simulink library "GenLib"  (R2019b)
settings: Solver=VariableStepAuto  StartTime=0.0  StopTime=10.0  RelTol=1e-3
undefined symbols (not defined in the file or in its folder): A, Ac, B, Bc, C, Cc, Dc, Dd, g, gcbh, I1_init, j, Mag_V0, np, nq, p, P0, PQext, Q0, sps_rtmsupport, Tp1, Tp2, Tq1, Tq2, Vbase, Vmin, Vnom
settings Model: Creator=haochen  LastModifiedBy=gdudgeon
settings DataIOCC: ReturnWorkspaceOutputs=off
settings OptimizationCC: LifeSpan=inf
settings DebuggingCC: SFExecutionAtInitializationDiag=none  ArithmeticOperatorsInVariantConditions=warning
settings SFSimCC: SimUseLocalCustomCode=off  CustomCodeUndefinedFunction=UseInterfaceOnly
settings RTWCC: RTWUseLocalCustomCode=off
settings CodeAppCC: StateflowObjectComments=on
settings ConfigComp: CovMetricSettings=dswe

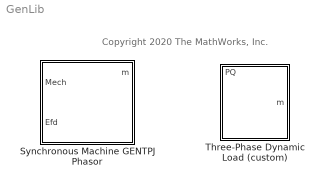
== system GenLib ==
  note: Copyright 2020 The MathWorks, Inc.
  Synchronous Machine GENTPJ Phasor : Subsystem  DialogController=POWERSYS.PowerSysDialog  LoadFcn=sps_rtmsupport('LoadFcn',gcbh);  StartFcn=sps_rtmsupport('StartFcn',gcbh);  StopFcn=sps_rtmsupport('StopFcn',gcbh);  mask(Synchronous Machine){PresetModel=No, MechanicalLoad=Mechanical power Pm, ShowDetailedParameters=on, RotorType=Salient-pole, Units=per unit fundamental parameters, MeasurementBus=off, NominalParameters=[ 187E6  13800   60], Stator=[ 2.85E-03  0.114  1.19  0.36 ], Field=[ 5.79E-04  0.114], Dampers2=[0.0652, 0.5134, 0.0287, 0.2553, 7.765e-3, 0.9167 ], Dampers1=[ 1.17E-02  0.182  1.97E-02  0.384 ], Mechanical=[ 3.7 0 20], PolePairs=20, InitialConditions=[ 0  0  0  0  0  0  0  0  1 ], SetSaturation=off, Saturation=[0.6404,0.7127,0.8441,0.9214,0.9956,1.082,1.19,1.316,1.457;0.7,0.7698,0.8872,0.9466,0.9969,1.046,1.1,1.151,1.201], LoadFlowParameters=[1,0,0,0,0], TsPowergui=0, TsBlock=-1, IterativeModel=Trapezoidal non iterative, IterativeDiscreteModel=Trapezoidal non iterative, BusType=PV, Pref=0, Qref=0, Qmin=-inf, Qmax=inf, PLF=0, QLF=0, Pnom=g.MBASE*1e6, Vnom=g.BUSV*1e3, fnom=60, Ra=p.ra, Xl=p.ll, Xd=p.ld, Xq=p.lq, Xdp=p.lpd, Xqp=p.lpq, Xdpp=p.lppd, Xqpp=p.lppq, Tdop=p.tpdo, Tqop=p.tpqo, Tdopp=p.tppdo, Tqopp=p.tppqo, SatOption=Quadratic, Ifd=[0 0.5 0.6 0.7 0.8 0.9 1 1.0562 1.1184 1.1985 1.2994 1.4576 1.6524 2.2234], Vag=[0 0.5 0.6 0.7 0.8 0.9 0.995 1.05 1.1 1.15 1.2 1.25 1.3 1.4], S10S12=[p.s1 p.s12], Kis=p.kis, SatOn=on, InputType=Mechanical power Pm, H=p.h, D=p.d}
      mask prompts: PresetModel "Preset  model:"; MechanicalLoad "Mechanical input:"; ShowDetailedParameters "Show detailed parameters"; RotorType "Rotor type:"; Units "Mask units:"; MeasurementBus "Use signal names to identify bus labels"; NominalParameters "Nominal power, line-to-line voltage and frequency [ Pn(VA)  Vn(Vrms)  fn(Hz) ]:"; Stator "Stator  [ Rs  Ll  Lmd  Lmq ] (pu):"; Field "Field  [ Rf  Llfd ] (pu):"; Dampers2 "Dampers  [ Rkd  Llkd  Rkq1  Llkq1  Rkq2  Llkq2 ] (pu):"; Dampers1 "Dampers  [ Rkd  Llkd  Rkq1  Llkq1 ] (pu):"; Mechanical "Inertia coeficient, friction factor, pole pairs [ H(s)  F(pu)  p() ]:"; PolePairs "Pole pairs p ():"; InitialConditions "Initial conditions [ dw(%)  th(deg)  ia,ib,ic(pu)  pha,phb,phc(deg)  Vf(pu) ]:"; SetSaturation "Simulate saturation"; Saturation "[ ifd; vt] (pu):"; LoadFlowParameters "Load Flow:   [Bus Type, Active Power,  UAB, phase of UAN ]"; TsPowergui "Sample time of powergui block:"; TsBlock "Sample time (-1 for inherited):"; IterativeDiscreteModel "Discrete solver model"; BusType "Generator type:"; Pref "Active power generation P (W):"; Qref "Reactive power generation Q (var):"; Qmin "Minimum reactive power Qmin (var):"; Qmax "Maximum reactive power Qmax (var):"; PLF "Load flow solution:  P_LF (W):"; QLF "Load flow solution:  Q_LF (var):"; Pnom "Nominal power (VA):"; Vnom "Nominal line-to-line voltage (Vrms):"; fnom "Nominal frequency (Hz):"; Ra "Stator resistance Ra:"; Xl "Stator leakage reactance Xl:"; Xd "d-axis reactance Xd:"; Xq "q-axis reactance Xq:"; Xdp "d-axis transient reactance Xd':"; Xqp "q-axis transient reactance Xq':"; Xdpp "d-axis subtransient reactance Xd'':"; Xqpp "q-axis subtransient reactance Xq'':"; Tdop "d-axis transient open-circuit time constant Tdo' (s):"; Tqop "q-axis transient open-circuit time constant Tqo' (s):"; Tdopp "d-axis subtransient open-circuit time constant Tdo''(s):"; Tqopp "q-axis subtransient open-circuit time constant Tqo''(s):"; SatOption "Option:"; Ifd "Field current saturation data (non-reciprocal pu):"; Vag "Air-gap voltage saturation data (pu):"; S10S12 "Saturation factors S10 and S12:"; SatOn "Simulate saturation"; InputType "Input type:"; H "Inertia constant H (s):"; D "damping coefficient D (pu):"
      mask help: Implements a 3-phase synchronous machine modelled in the dq rotor reference frame. Stator windings are connected in wye to an internal neutral point.
      mask init:
      | %block = gcb;
      | %[Ts,SM,WantBlockChoice,X,Y] = powericon('SynchronousMachineInit',block,TsPowergui,TsBlock,MechanicalLoad,Units,RotorType,NominalParameters,Mechanical,PolePairs,InitialConditions,SetSaturation,Saturation,IterativeModel,MeasurementBus,Stator,Field,Dampers1,Dampers2);
      | %powericon('SetInternalModels','set',block,WantBlockChoice); sps_rtmsupport('parametereditingmodes',block, [1 2 3 4 5 6 15 20 21 22]); 
      | %powericon('ShaftInput',block);
      | 
      | powericon('psbloadfunction',gcb,'gotofrom','UpdateGotoTag');
      | 
      | % base values
      | Pbase = Pnom;                 % base power
      | Vbase = Vnom/sqrt(3)*sqrt(2); % base voltage, line-neutral, peak value
      | Ibase = Pbase/(1.5*Vbase);    % base curretn, peak value
      | wbase = 2*pi*fnom;            % base radial frequency
      | 
      | % saturation
      | switch SatOption
      |     case 'Saturation data (i.e., field current vs. air-gap voltage)'
      |         xVec = 0:0.1:1.5;
      |         IfnrVec = interp1(Vag, Ifd, xVec, 'linear', 'extrap');
      |         SatX = (IfnrVec - xVec)./xVec;
      |         SatX(1) = 0;
      |         
      |     otherwise
      |         S10 = S10S12(1);
      |         S12 = S10S12(2);
      |         if S10<0 || S12<0
      |             error('S10 and S12 should be non-negative values.');
      |         end
      |         if S10 >= S12
      |             error('S10 should be less than S12.');
      |         end
      |         
      |         switch SatOption  
      |             case 'Quadratic'
      |                 AVec = [ (300*S10 - 250*S12 + 50*(S10*S12)^(1/2))/(250*S10 - 250*S12);...
      |                         -(250*S12 - 300*S10 + 50*(S10*S12)^(1/2))/(250*S10 - 250*S12) ];
      |                 BVec = [ 25*S10 + 25*S12 - 50*(S10*S12)^(1/2);...
      |                          25*S10 + 25*S12 + 50*(S10*S12)^(1/2) ];
      |                 A = min(AVec);
      |                 B = unique(BVec(AVec==A));
      |                 if A < 0
      |                     error('A is negative. The specified S10 and S12 cannot make the saturation curve pass the origin point.');
      |                 end
      |                 % xVec = A:(1.5-A)/10:1.5;
      |                 xVec = A:(10-A)/100:10;
      |                 SatX = B*(xVec-A).^2;
      |                 xVec = [0, xVec];
      |                 SatX = [0, SatX];
      |                 
      |             case 'Scaled Quadratic' 
      |                 AVec = [ (300*S10 - 300*S12 + 10*30^(1/2)*(S10*S12)^(1/2))/(250*S10 - 300*S12);...
      |                         -(300*S12 - 300*S10 + 10*30^(1/2)*(S10*S12)^(1/2))/(250*S10 - 300*S12) ];
      |                 BVec = [ 25*S10 + 30*S12 - 10*30^(1/2)*(S10*S12)^(1/2);...
      |                          25*S10 + 30*S12 + 10*30^(1/2)*(S10*S12)^(1/2) ];
      |                 A = min(AVec);
      |                 B = unique(BVec(AVec==A));
      |                 if A < 0
      |                     error('A is negative. The specified S10 and S12 cannot make the saturation curve pass the origin point.');
      |                 end
      |                 xVec = A:(1.5-A)/10:1.5;
      |                 SatX = B*(xVec-A).^2./xVec;
      |                 xVec = [0, xVec];
      |                 SatX = [0, SatX];
      |                 
      |             case 'Exponential'
      |                 if S10 == 0
      |                     error('S10 cannot be zero for the exponential function.');
      |                 else
      |                     A = log(S10/S12)/log(1/1.2);
      |                     B = S10;
      |                 end;
      |                 xVec = 0:0.05:1.5;
      |                 SatX = B*(xVec).^A;
      |         end
      |       
      | end
      | 
      | switch InputType
      |     case 'Mechanical power Pm'
      |         set_param([gcb '/Mechanical model'],'OverrideUsingVariant','PmIn');
      |     otherwise
      |         set_param([gcb '/Mechanical model'],'OverrideUsingVariant','wIn');
      | end
      settings: CopyFcn=sps_rtmsupport('CopyFcn',gcbh); powericon('psbloadfunction',gcb,'gotofrom','UpdateGotoTag');  DeleteFcn=sps_rtmsupport('DeleteFcn',gcbh);  UndoDeleteFcn=sps_rtmsupport('UndoDeleteFcn',gcbh);  ModelCloseFcn=sps_rtmsupport('ModelCloseFcn',gcbh);  PreSaveFcn=sps_rtmsupport('PreSaveFcn',gcbh);  PostSaveFcn=sps_rtmsupport('PostSaveFcn',gcbh);  NameChangeFcn=sps_rtmsupport('NameChangeFcn',gcbh);  PreCopyFcn=sps_rtmsupport('PreCopyFcn',gcbh);  CloseFcn=sps_rtmsupport('CloseFcn',gcbh);  PreDeleteFcn=sps_rtmsupport('PreDeleteFcn',gcbh);
      mask Help: helpview(psbhelp);
      mask TypeOptions PresetModel: No | 01: 50Hz 400V 8.1kVA 1500RPM | 02: 50Hz 400V 16kVA 1500RPM | 03: 50Hz 400V 31.3kVA 1500RPM | 04: 50Hz 400V 42.5kVA 1500RPM | 05: 50Hz 400V 60kVA 1500RPM | 06: 50Hz 400V 85kVA 1500RPM | 07: 50Hz 400V 250kVA 1500RPM | 08: 50Hz 400V 325kVA 1500RPM | 09: 50Hz 400V 670kVA 1500RPM | 10: 50Hz 400V 910kVA 1500RPM | 11: 50Hz 400V 1320kVA 1500RPM | 12: 50Hz 400V 2000kVA 1500RPM | 13: 60Hz 460V 10.2kVA 1800RPM | 14: 60Hz 460V 20kVA 1800RPM | 15: 60Hz 460V 37.5kVA 1800RPM | 16: 60Hz 460V 52.5kVA 1800RPM | 17: 60Hz 460V 72.5kVA 1800RPM | 18: 60Hz 460V 100kVA 1800RPM | 19: 60Hz 460V 300kVA 1800RPM | 20: 60Hz 460V 406kVA 1800RPM | 21: 60Hz 460V 800kVA 1800RPM | 22: 60Hz 460V 1075kVA 1800RPM | 23: 60Hz 460V 1588kVA 1800RPM | 24: 60Hz 460V 2500kVA 1800RPM
      mask Callback PresetModel: powericon('SynchronousMachineCback',gcb,'per unit fundamental parameters');
      mask TypeOptions MechanicalLoad: Mechanical power Pm | Speed w | Mechanical rotational port
      mask Callback MechanicalLoad: powericon('SynchronousMachineCback',gcb,'per unit fundamental parameters');
      mask Callback ShowDetailedParameters: %powericon('SynchronousMachineCback',gcb,'per unit fundamental parameters');
      mask TypeOptions RotorType: Salient-pole | Round
      mask Callback RotorType: powericon('SynchronousMachineCback',gcb,'per unit fundamental parameters');
      mask TypeOptions Units: per unit fundamental parameters
      mask Callback SetSaturation: powericon('SynchronousMachineCback',gcb,'per unit fundamental parameters');
      mask TypeOptions IterativeModel: Trapezoidal non iterative | Trapezoidal iterative (alg. loop) | Forward Euler
      mask TypeOptions IterativeDiscreteModel: Trapezoidal non iterative | Trapezoidal iterative (alg. loop)
      mask TypeOptions BusType: swing | PV | PQ
      mask Callback BusType: powericon('SynchronousMachineCback',gcb,'per unit fundamental parameters');
      mask Callback QLF: sps_rtmsupport('parametereditingmodes',gcbh, [1 2 3 4 5 6 15 20 21 22]);
      mask TypeOptions SatOption: Saturation data (i.e., field current vs. air-gap voltage) | Quadratic | Scaled Quadratic | Exponential
      mask Callback SatOption:
      | switch get_param(gcb,'SatOption')
      |     case 'Saturation data (i.e., field current vs. air-gap voltage)'
      |         switch get_param(gcb,'InputType')
      |             case 'Mechanical power Pm'
      |                 set_param(gcb,'MaskVisibilities',{'off';'off';'off';'off';'off';'off';'off';'off';'off';'off';'off';'off';'off';'off';'off';'off';'off';'off';'off';'off';'off';'off';'off';'off';'off';'off';'off';'off';...
      |                     'on';'on';'on';  'on';'on';'on';'on';  'on';'on';'on';'on';  'on';'on';'on';'on';'on';  'on';'on';'off';'on';'on';  'on';'on';'on'})
      |             otherwise
      |                 set_param(gcb,'MaskVisibilities',{'off';'off';'off';'off';'off';'off';'off';'off';'off';'off';'off';'off';'off';'off';'off';'off';'off';'off';'off';'off';'off';'off';'off';'off';'off';'off';'off';'off';...
      |                     'on';'on';'on';  'on';'on';'on';'on';  'on';'on';'on';'on';  'on';'on';'on';'on';'on';  'on';'on';'off';'on';'on';  'on';'off';'off'})
      |         end
      |     otherwise
      |         switch get_param(gcb,'InputType')
      |             case 'Mechanical power Pm'
      |                 set_param(gcb,'MaskVisibilities',{'off';'off';'off';'off';'off';'off';'off';'off';'off';'off';'off';'off';'off';'off';'off';'off';'off';'off';'off';'off';'off';'off';'off';'off';'off';'off';'off';'off';...
      |                     'on';'on';'on';  'on';'on';'on';'on';  'on';'on';'on';'on';  'on';'on';'on';'on';'on';  'off';'off';'on';'on';'on';  'on';'on';'on'})
      |             otherwise
      |                 set_param(gcb,'MaskVisibilities',{'off';'off';'off';'off';'off';'off';'off';'off';'off';'off';'off';'off';'off';'off';'off';'off';'off';'off';'off';'off';'off';'off';'off';'off';'off';'off';'off';'off';...
      |                     'on';'on';'on';  'on';'on';'on';'on';  'on';'on';'on';'on';  'on';'on';'on';'on';'on';  'off';'off';'on';'on';'on';  'on';'off';'off'})
      |         end
      | 
      | end
      mask TypeOptions InputType: Mechanical power Pm | Speed w
      mask Callback InputType:
      | switch get_param(gcb,'SatOption')
      |     case 'Saturation data (i.e., field current vs. air-gap voltage)'
      |         switch get_param(gcb,'InputType')
      |             case 'Mechanical power Pm'
      |                 set_param(gcb,'MaskVisibilities',{'off';'off';'off';'off';'off';'off';'off';'off';'off';'off';'off';'off';'off';'off';'off';'off';'off';'off';'off';'off';'off';'off';'off';'off';'off';'off';'off';'off';...
      |                     'on';'on';'on';  'on';'on';'on';'on';  'on';'on';'on';'on';  'on';'on';'on';'on';'on';  'on';'on';'off';'on';'on';  'on';'on';'on'})
      |             otherwise
      |                 set_param(gcb,'MaskVisibilities',{'off';'off';'off';'off';'off';'off';'off';'off';'off';'off';'off';'off';'off';'off';'off';'off';'off';'off';'off';'off';'off';'off';'off';'off';'off';'off';'off';'off';...
      |                     'on';'on';'on';  'on';'on';'on';'on';  'on';'on';'on';'on';  'on';'on';'on';'on';'on';  'on';'on';'off';'on';'on';  'on';'off';'off'})
      |         end
      |     otherwise
      |         switch get_param(gcb,'InputType')
      |             case 'Mechanical power Pm'
      |                 set_param(gcb,'MaskVisibilities',{'off';'off';'off';'off';'off';'off';'off';'off';'off';'off';'off';'off';'off';'off';'off';'off';'off';'off';'off';'off';'off';'off';'off';'off';'off';'off';'off';'off';...
      |                     'on';'on';'on';  'on';'on';'on';'on';  'on';'on';'on';'on';  'on';'on';'on';'on';'on';  'off';'off';'on';'on';'on';  'on';'on';'on'})
      |             otherwise
      |                 set_param(gcb,'MaskVisibilities',{'off';'off';'off';'off';'off';'off';'off';'off';'off';'off';'off';'off';'off';'off';'off';'off';'off';'off';'off';'off';'off';'off';'off';'off';'off';'off';'off';'off';...
      |                     'on';'on';'on';  'on';'on';'on';'on';  'on';'on';'on';'on';  'on';'on';'on';'on';'on';  'off';'off';'on';'on';'on';  'on';'off';'off'})
      |         end
      | 
      | end
      mask DialogControl Container4 Prompt: Configuration
      mask DialogControl Container9 Prompt: Measurement output
      mask DialogControl Container6 Prompt: Parameters
      mask DialogControl PlotSaturation Prompt: Plot
      mask DialogControl PlotSaturation Callback:
      | Saturation = evalin('base',get_param(gcbh,'Saturation'));
      | figure;plot(Saturation(1,:),Saturation(2,:),'*-');
      | xlabel(['ifd =', mat2str(Saturation(1,:),4)]);
      | ylabel(['vt =', mat2str(Saturation(2,:),4)]);
      mask DialogControl Container12 Prompt: Advanced
      mask DialogControl Control3 Prompt: Discrete solver model:
      mask DialogControl Control5 Prompt: This solver model is not recommended.
      mask DialogControl Control6 Prompt: Why?
      mask DialogControl Control6 Callback: web(fullfile(docroot, 'physmod/sps/powersys/ref/synchronousmachine.html#zmw57dd0e55004'))
      mask DialogControl Container7 Prompt: Load Flow
      mask DialogControl Container13 Prompt: Main
      mask DialogControl Container14 Prompt: Impedances (per unit)
      mask DialogControl Container15 Prompt: Time constants (s)
      mask DialogControl Container16 Prompt: Saturation
      mask DialogControl Container17 Prompt: Mechanical
      mask Display:
      | %plot(X.p1,Y.p1,X.p2,Y.p2,X.p3,Y.p3,X.p4,Y.p4,X.p5,Y.p5,X.p6,Y.p6,X.p7,Y.p7)
      | %color('blue');
      | %plot(X.p8,Y.p8)
      | %plot(X.p9,Y.p9)
      | %port_label('input',1,SM.PortLabel)
  Three-Phase Dynamic Load (custom) : Subsystem  DialogController=POWERSYS.PowerSysDialog  LoadFcn=sps_rtmsupport('LoadFcn',gcbh);  StartFcn=sps_rtmsupport('StartFcn',gcbh);  StopFcn=sps_rtmsupport('StopFcn',gcbh);  mask(Three-Phase Dynamic Load){NominalVoltage=[ 230e3 60 ], ActiveReactivePowers=[0 0], PositiveSequence=[1 0], ExternalControl=on, NpNq=[1.3 2], TimeConstants=[0  0  0  0], MinimumVoltage=0.7, LoadFlowParameters=[4,0,0,0,0]}
      mask prompts: NominalVoltage "Nominal L-L voltage and frequency  [Vn(Vrms) fn(Hz)]:"; ActiveReactivePowers "Active and reactive power at initial voltage [Po(W) Qo(var)]:"; PositiveSequence "Initial positive-sequence voltage Vo [Mag(pu) Phase (deg.)]:"; ExternalControl "External control of PQ"; NpNq "Parameters [ np  nq ]:"; TimeConstants "Time constants [Tp1 Tp2 Tq1 Tq2]  (s):"; MinimumVoltage "Minimum voltage Vmin (pu):"; LoadFlowParameters "Load Flow parameters"
      mask help:
      | Implements a three-phase, three-wire dynamic load. Active  power P and reactive
      |  power Q absorbed by the load vary as function of positive-sequence voltage V
      | according to following equations:
      |
      |   If V>Vmin, P and Q vary as follows:
      |        P=Po*(V/Vo)^np*(1+Tp1.s)/(1+Tp2.s)
      |        Q=Qo*(V/Vo)^nq*(1+Tq1.s)/(1+Tq2.s)
      |   if V<Vmin
      |      Same equations with np=nq=2 (constant impedance load)
      |
      | Check 'External control of PQ'  to control power from a vectorized Simulink
      | signal  [P Q] .
      mask init:
      | block = gcb;
      | [Ts, WantBlockChoice, Vnom,fnom,P0,Q0,Mag_V0,Pha_V0,V0_d,V0_q,np,nq,Tp1,Tp2,Tq1,Tq2,Vbase,I1_init,Mag_ia,Phase_ia,Vmin,PQext,a] = powericon('ThreePhaseDynamicLoadInit',block,NominalVoltage,ActiveReactivePowers,PositiveSequence,NpNq,TimeConstants,MinimumVoltage,ExternalControl);
      | % powericon('SetInternalModels','set',block,WantBlockChoice);
      settings: CopyFcn=sps_rtmsupport('CopyFcn',gcbh); powericon('psbloadfunction',gcb,'gotofrom','UpdateGotoTag');  DeleteFcn=sps_rtmsupport('DeleteFcn',gcbh);  UndoDeleteFcn=sps_rtmsupport('UndoDeleteFcn',gcbh);  ModelCloseFcn=sps_rtmsupport('ModelCloseFcn',gcbh);  PreSaveFcn=sps_rtmsupport('PreSaveFcn',gcbh);  PostSaveFcn=sps_rtmsupport('PostSaveFcn',gcbh);  NameChangeFcn=sps_rtmsupport('NameChangeFcn',gcbh);  PreCopyFcn=sps_rtmsupport('PreCopyFcn',gcbh);  OpenFcn=sps_rtmsupport('OpenFcn',gcbh, 4);  CloseFcn=sps_rtmsupport('CloseFcn',gcbh);  PreDeleteFcn=sps_rtmsupport('PreDeleteFcn',gcbh);
      mask Help: helpview(psbhelp)
      mask Callback ExternalControl: %powericon('ThreePhaseDynamicLoadCback',gcb);
      mask Display:
      | plot(-45,-45,45,45,[0,9,18,24,29,30,29,24,18,9,0,-9,-18,-24,-29,-30,-29,-24,-18,-9,0]*.9,[30,29,24,18,9,0,-9,-18,-24,-29,-30,-29,-24,-18,-9,0,9,18,24,29,30]*.9)
      | plot([0,0,10,0,-10,0]*1.1,[15,-5,-5,-15,-5,-5]*1.1)

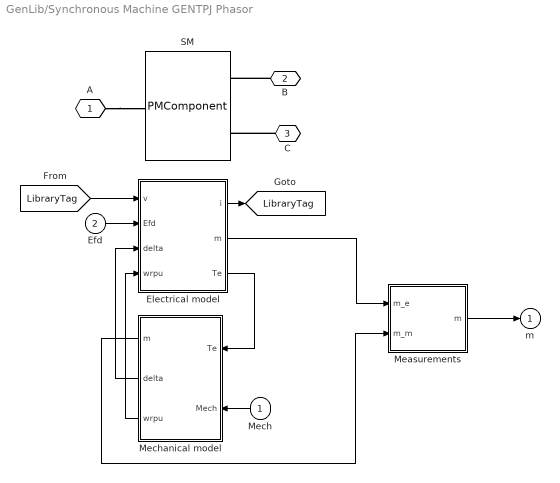
== system GenLib/Synchronous Machine GENTPJ Phasor ==
  Mech : Inport
  Efd : Inport  Port=2
  Electrical model : Subsystem
  Measurements : Subsystem
  Mechanical model : Subsystem  VariantControlMode=Label  Variant=on  LabelModeActiveChoice=PmIn
  SM : PMComponent  PhysicalDomain=powersysdomain  LeftPortType=p1  RightPortType=p1  LConnTagsString=__newl0  RConnTagsString=B|C  mask(InnerPowersysBlock){}
  A : PMIOPort  Side=Right
  B : PMIOPort  Port=2  Side=Right
  C : PMIOPort  Port=3  Side=Right
  m : Outport  InitialOutput=0  VectorParamsAs1DForOutWhenUnconnected=off
  tag scope: LibraryTag=global
  wires:
  [LibraryTag] -> Electrical model/1(v)
  Measurements/1(m) -> m/1
  Electrical model/3(Te) -> Mechanical model/1(Te)
  Mechanical model/1(m) -> Measurements/2(m_m)
  Electrical model/2(m) -> Measurements/1(m_e)
  Mech/1 -> Mechanical model/2(Mech)
  Electrical model/1(i) -> [LibraryTag]
  Efd/1 -> Electrical model/2(Efd)
  Mechanical model/2(delta) -> Electrical model/3(delta)
  Mechanical model/3(wrpu) -> Electrical model/4(wrpu)
  connections:
  A/RConn1 -- SM/LConn1
  B/RConn1 -- SM/RConn1
  C/RConn1 -- SM/RConn2

== system GenLib/Three-Phase Dynamic Load (custom) ==
  PQ : Inport
  3-PhaseDynamicLoad : PMComponent  PhysicalDomain=powersysdomain  LeftPortType=p1  RightPortType=p1  LConnTagsString=A|B  RConnTagsString=C  mask(InnerPowersysBlock){}
  Measurement list : Subsystem
  Model : Subsystem
  A : PMIOPort  Side=Left
  B : PMIOPort  Port=2  Side=Left
  C : PMIOPort  Port=3  Side=Left
  m : Outport  InitialOutput=[0,0,0]  VectorParamsAs1DForOutWhenUnconnected=off
  tag scope: LibraryTag=global
  wires:
  Measurement list/1(Out1) -> m/1
  Model/1(i) -> [LibraryTag]
  [LibraryTag] -> Model/1(v)
  Model/2(m) -> Measurement list/1(In1)
  PQ/1 -> Model/2(PQ)
  connections:
  A/RConn1 -- 3-PhaseDynamicLoad/LConn1
  B/RConn1 -- 3-PhaseDynamicLoad/LConn2
  C/RConn1 -- 3-PhaseDynamicLoad/RConn1

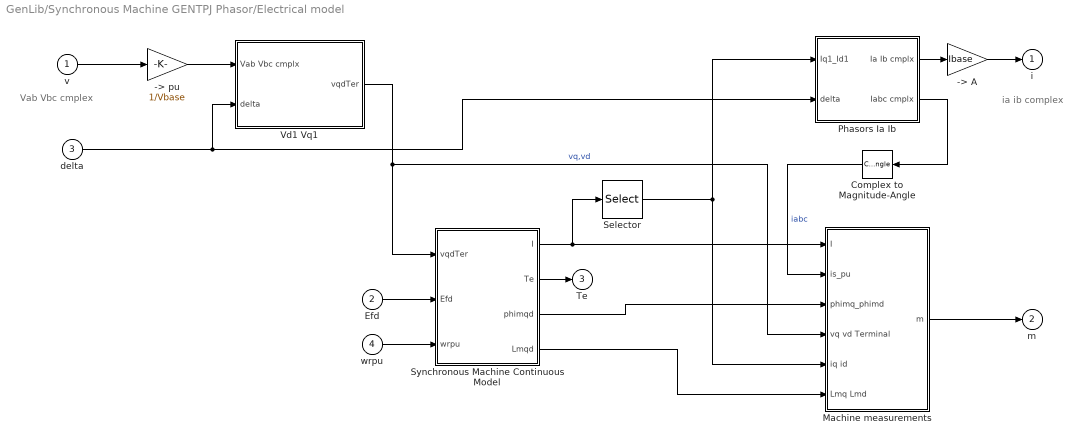
== system GenLib/Synchronous Machine GENTPJ Phasor/Electrical model ==
  note: ia ib complex
  note: Vab Vbc cmplex
  v : Inport
  Efd : Inport  Port=2
  delta : Inport  Port=3
  wrpu : Inport  Port=4  PortDimensions=1
  -> A : Gain  Gain=Ibase
  -> pu : Gain  Gain=1/Vbase
  Complex to Magnitude-Angle : ComplexToMagnitudeAngle  Output=Magnitude
  Machine measurements : Subsystem
  Phasors Ia Ib : Subsystem
  Selector : Selector  InputPortWidth=3  IndexOptions=Index vector (dialog)  Indices=[1 2]  OutputSizes=1
  Synchronous Machine Continuous Model : Subsystem
  Vd1 Vq1 : Subsystem
  i : Outport  InitialOutput=0  VectorParamsAs1DForOutWhenUnconnected=off
  m : Outport  Port=2  InitialOutput=0  VectorParamsAs1DForOutWhenUnconnected=off
  Te : Outport  Port=3  InitialOutput=0  VectorParamsAs1DForOutWhenUnconnected=off
  wires:
  Efd/1 -> Synchronous Machine Continuous Model/2(Efd)
  wrpu/1 -> Synchronous Machine Continuous Model/3(wrpu)
  -> pu/1 -> Vd1 Vq1/1(Vab Vbc cmplx)
  v/1 -> -> pu/1
  Phasors Ia Ib/1(Ia Ib cmplx) -> -> A/1
  -> A/1 -> i/1
  Phasors Ia Ib/2(Iabc cmplx) -> Complex to Magnitude-Angle/1
  Complex to Magnitude-Angle/1 -> Machine measurements/2(is_pu)  "iabc"
  Synchronous Machine Continuous Model/1(I) -> Selector/1, Machine measurements/1(I)
  Selector/1 -> Phasors Ia Ib/1(Iq1_Id1), Machine measurements/5(iq id)
  Synchronous Machine Continuous Model/2(Te) -> Te/1
  Synchronous Machine Continuous Model/3(phimqd) -> Machine measurements/3(phimq_phimd)
  delta/1 -> Vd1 Vq1/2(delta), Phasors Ia Ib/2(delta)
  Vd1 Vq1/1(vqdTer) -> Synchronous Machine Continuous Model/1(vqdTer), Machine measurements/4(vq vd Terminal)  "vq,vd"
  Synchronous Machine Continuous Model/4(Lmqd) -> Machine measurements/6(Lmq Lmd)
  Machine measurements/1(m) -> m/1

== system GenLib/Synchronous Machine GENTPJ Phasor/Measurements ==
  m_e : Inport
  m_m : Inport  Port=2
  Bus Creator1 : BusCreator  Inputs="'Stator current','dq0 components','Mechanical','Load angle   delta  (deg)','Output active power   Peo (pu)','Output reactive power  Qeo (pu)'"
  Bus Creator2 : BusCreator  Inputs=3
  Bus Creator3 : BusCreator  Inputs=9
  Bus Creator4 : BusCreator  Inputs=5
  Demux : Demux  Outputs=15
  Demux1 : Demux  Outputs=[1,1,1,1,1]
  m : Outport  VectorParamsAs1DForOutWhenUnconnected=off
  wires:
  Demux1/5 -> Bus Creator4/5  "Electromagnetic torque  Te (pu)"
  Demux/12 -> Bus Creator3/9  "Lmd (pu)"
  Demux/11 -> Bus Creator3/8  "Lmq (pu)"
  Demux/10 -> Bus Creator3/7  "Stator voltage  vd (pu)"
  Demux/9 -> Bus Creator3/6  "Stator voltage  vq (pu)"
  Demux/8 -> Bus Creator3/5  "Mutual flux  phimd (pu)"
  Demux/7 -> Bus Creator3/4  "Mutual flux  phimq (pu)"
  Demux/13 -> Bus Creator1/4  "Load angle   delta  (deg)"
  Demux/14 -> Bus Creator1/5  "Output active power   Peo (pu)"
  Demux/15 -> Bus Creator1/6  "Output reactive power  Qeo (pu)"
  Demux1/4 -> Bus Creator4/4  "Rotor speed deviation  dwr (pu)"
  Demux1/3 -> Bus Creator4/3  "Electrical power  Pe (pu)"
  Demux1/2 -> Bus Creator4/2  "Rotor speed  wm  (pu)"
  Demux1/1 -> Bus Creator4/1  "Rotor angle deviation  delta (rad)"
  m_m/1 -> Demux1/1
  m_e/1 -> Demux/1
  Bus Creator1/1 -> m/1
  Demux/1 -> Bus Creator2/1  "is_a (pu)"
  Demux/2 -> Bus Creator2/2  "is_b (pu)"
  Demux/3 -> Bus Creator2/3  "is_c (pu)"
  Bus Creator2/1 -> Bus Creator1/1  "Stator current"
  Demux/4 -> Bus Creator3/1  "Stator current  iq (pu)"
  Demux/5 -> Bus Creator3/2  "Stator current  id (pu)"
  Demux/6 -> Bus Creator3/3  "Field current  ifd (pu)"
  Bus Creator3/1 -> Bus Creator1/2  "dq0 components"
  Bus Creator4/1 -> Bus Creator1/3  "Mechanical"

== system GenLib/Synchronous Machine GENTPJ Phasor/Mechanical model ==
  Te : Inport
  Mech : Inport  Port=2
  Pm input : Subsystem  VariantControl=PmIn
  w input : Subsystem  VariantControl=wIn
  m : Outport  VectorParamsAs1DForOutWhenUnconnected=off
  delta : Outport  Port=2  VectorParamsAs1DForOutWhenUnconnected=off
  wrpu : Outport  Port=3  VectorParamsAs1DForOutWhenUnconnected=off

== system GenLib/Three-Phase Dynamic Load (custom)/Measurement list ==
  In1 : Inport
  Bus Creator1 : BusCreator  Inputs=3
  Demux : Demux  Outputs=[1,1,1]
  Out1 : Outport  VectorParamsAs1DForOutWhenUnconnected=off
  wires:
  In1/1 -> Demux/1
  Bus Creator1/1 -> Out1/1
  Demux/2 -> Bus Creator1/2  "Active power P (W)"
  Demux/1 -> Bus Creator1/1  "Positive-sequence voltage V (pu)"
  Demux/3 -> Bus Creator1/3  "Reactive power Q (var)"

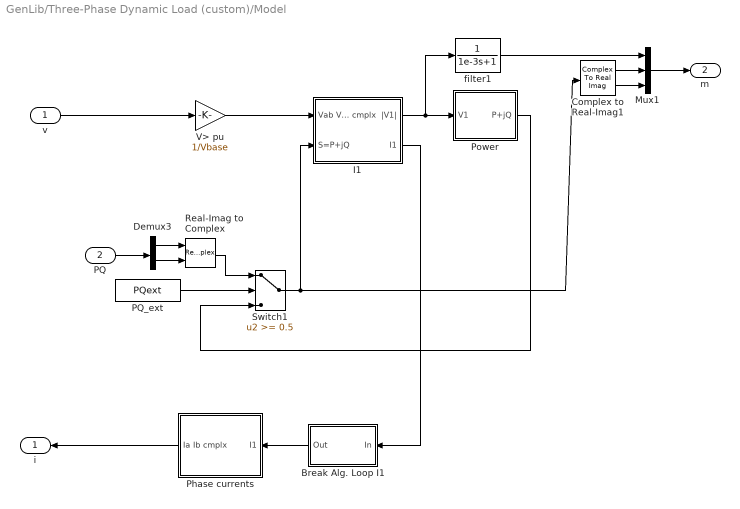
== system GenLib/Three-Phase Dynamic Load (custom)/Model ==
  v : Inport
  PQ : Inport  Port=2
  " filter1" : TransferFcn  Denominator=[1e-3 1]
  Break Alg. Loop I1 : Subsystem
  Complex to Real-Imag1 : ComplexToRealImag
  Demux3 : Demux  Outputs=2
  "I1 " : Subsystem
  Mux1 : Mux  Inputs=3
  PQ_ext : Constant  Value=PQext
  Phase currents : Subsystem
  Power : Subsystem
  Real-Imag to Complex : RealImagToComplex
  Switch1 : Switch  Threshold=0.5  InputSameDT=on
  V> pu : Gain  Gain=1/Vbase  SaturateOnIntegerOverflow=on  OutDataTypeStr=Inherit: Same as input  ParamDataTypeStr=Inherit: Same as input
  i : Outport  VectorParamsAs1DForOutWhenUnconnected=off
  m : Outport  Port=2  VectorParamsAs1DForOutWhenUnconnected=off
  wires:
  Phase currents/1(Ia Ib cmplx) -> i/1
  Power/1(P+jQ) -> Switch1/3
  Break Alg. Loop I1/1(Out) -> Phase currents/1(I1)
  v/1 -> V> pu/1
  "I1 "/1(|V1|) -> " filter1"/1, Power/1(V1)
  V> pu/1 -> "I1 "/1(Vab Vbc cmplx)
  "I1 "/2(I1) -> Break Alg. Loop I1/1(In)
  " filter1"/1 -> Mux1/1
  Mux1/1 -> m/1
  Complex to Real-Imag1/1 -> Mux1/2
  Complex to Real-Imag1/2 -> Mux1/3
  PQ_ext/1 -> Switch1/2
  Switch1/1 -> "I1 "/2(S=P+jQ), Complex to Real-Imag1/1
  Real-Imag to Complex/1 -> Switch1/1
  Demux3/1 -> Real-Imag to Complex/1
  Demux3/2 -> Real-Imag to Complex/2
  PQ/1 -> Demux3/1

== system GenLib/Synchronous Machine GENTPJ Phasor/Electrical model/Machine measurements ==
  I : Inport
  is_pu : Inport  Port=2
  phimq_phimd : Inport  Port=3
  vq vd Terminal : Inport  Port=4
  iq id : Inport  Port=5
  Lmq Lmd : Inport  Port=6
  Delta angle : Subsystem
  Machine measurements : Mux  Inputs="[ 3 5 2  2  1 1 1]"
  Mux3 : Mux  Inputs=[3 2]
  PQ : Subsystem
  m : Outport  VectorParamsAs1DForOutWhenUnconnected=off
  wires:
  Lmq Lmd/1 -> Machine measurements/4  "Lmq,Lmd"
  iq id/1 -> PQ/1(Iqd)
  Machine measurements/1 -> m/1
  phimq_phimd/1 -> Mux3/2
  is_pu/1 -> Machine measurements/1
  vq vd Terminal/1 -> Machine measurements/3, PQ/2(Vqd), Delta angle/1(Vqd)  "Vq, Vd"
  PQ/2(Qeo) -> Machine measurements/7  "Qeo"
  PQ/1(Peo) -> Machine measurements/6  "Peo"
  Delta angle/1(delta) -> Machine measurements/5  "delta"
  Mux3/1 -> Machine measurements/2  "iq,id,ifd,phimq,phimd"
  I/1 -> Mux3/1  "iq, id, ifd"

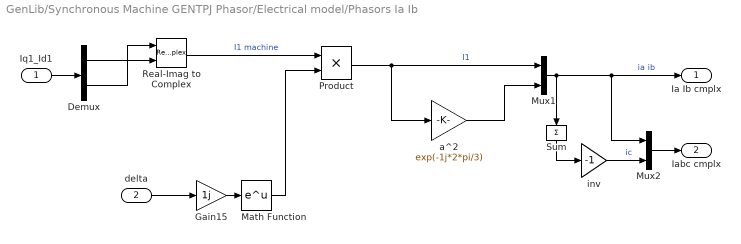
== system GenLib/Synchronous Machine GENTPJ Phasor/Electrical model/Phasors Ia Ib ==
  Iq1_Id1 : Inport  PortDimensions=2
  delta : Inport  Port=2
  Demux : Demux  Outputs=2
  Gain15 : Gain  Gain=1j  SaturateOnIntegerOverflow=on  OutDataTypeStr=Inherit: Same as input  ParamDataTypeStr=Inherit: Same as input
  Math Function : Math  SaturateOnIntegerOverflow=on
  Mux1 : Mux  Inputs=2
  Mux2 : Mux  Inputs=[2 1]
  Product : Product  SaturateOnIntegerOverflow=on  InputSameDT=on  OutDataTypeStr=Inherit: Same as first input
  Real-Imag to Complex : RealImagToComplex
  Sum : Sum  Inputs=1  SaturateOnIntegerOverflow=on  InputSameDT=on  OutDataTypeStr=Inherit: Same as first input
  a^2 : Gain  Gain=exp(-1j*2*pi/3)  SaturateOnIntegerOverflow=on  OutDataTypeStr=Inherit: Same as input  ParamDataTypeStr=Inherit: Same as input
  inv : Gain  Gain=-1  SaturateOnIntegerOverflow=on  OutDataTypeStr=Inherit: Same as input  ParamDataTypeStr=Inherit: Same as input
  Ia Ib cmplx : Outport  VectorParamsAs1DForOutWhenUnconnected=off
  Iabc cmplx : Outport  Port=2  VectorParamsAs1DForOutWhenUnconnected=off
  wires:
  delta/1 -> Gain15/1
  a^2/1 -> Mux1/2
  Demux/2 -> Real-Imag to Complex/1
  Demux/1 -> Real-Imag to Complex/2
  Product/1 -> Mux1/1, a^2/1  "I1"
  Iq1_Id1/1 -> Demux/1
  Mux1/1 -> Sum/1, Ia Ib cmplx/1, Mux2/1  "ia ib"
  Sum/1 -> inv/1
  inv/1 -> Mux2/2  "ic"
  Mux2/1 -> Iabc cmplx/1
  Gain15/1 -> Math Function/1
  Math Function/1 -> Product/2
  Real-Imag to Complex/1 -> Product/1  "I1 machine"

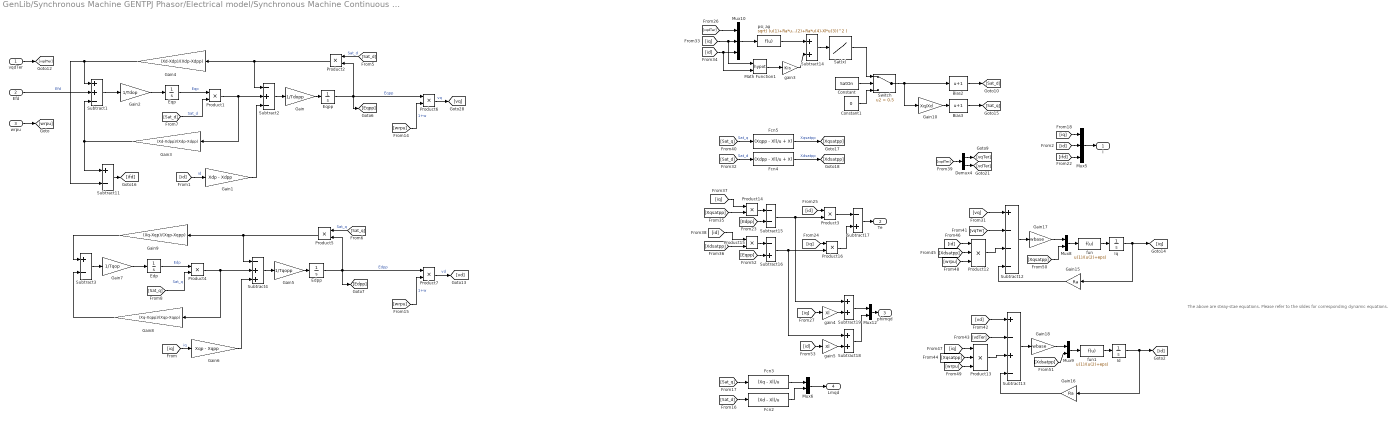
== system GenLib/Synchronous Machine GENTPJ Phasor/Electrical model/Synchronous Machine Continuous Model ==
  note: The above are steay-stae equations.
      | Please refer to the sildes for corresponding dynamic equations.
  vqdTer : Inport
  Efd : Inport  Port=2
  wrpu : Inport  Port=3
  Bias2 : Bias  Bias=1
  Bias3 : Bias  Bias=1
  Constant : Constant  Value=SatOn
  Constant1 : Constant  Value=0
  Demux4 : Demux  Outputs=2
  Edp : Integrator
  Edpp : Integrator
  Eqp : Integrator
  Eqpp : Integrator
  Fcn2 : Fcn  Expr=(Xd - Xl)/u
  Fcn3 : Fcn  Expr=(Xq - Xl)/u
  Fcn4 : Fcn  Expr=(Xdpp - Xl)/u + Xl
  Fcn5 : Fcn  Expr=(Xqpp - Xl)/u + Xl
  Gain : Gain  Gain=1/Tdopp
  Gain1 : Gain  Gain=Xdp - Xdpp
  Gain10 : Gain  Gain=Xq/Xd
  Gain15 : Gain  Gain=Ra
  Gain16 : Gain  Gain=Ra
  Gain17 : Gain  Gain=wbase
  Gain18 : Gain  Gain=wbase
  Gain2 : Gain  Gain=1/Tdop
  Gain3 : Gain  Gain=(Xd-Xdpp)/(Xdp-Xdpp)
  Gain4 : Gain  Gain=(Xd-Xdp)/(Xdp-Xdpp)
  Gain5 : Gain  Gain=1/Tqopp
  Gain6 : Gain  Gain=Xqp - Xqpp
  Gain7 : Gain  Gain=1/Tqop
  Gain8 : Gain  Gain=(Xq-Xqpp)/(Xqp-Xqpp)
  Gain9 : Gain  Gain=(Xq-Xqp)/(Xqp-Xqpp)
  Id : Integrator
  Iq : Integrator
  Math Function1 : Math  Operator=hypot  SaturateOnIntegerOverflow=on
  Mux10 : Mux  Inputs=3
  Mux{6,8..9,12} (4 alike) : Mux  Inputs=2
  Mux5 : Mux  Inputs=3
  Product{1..7,14..16} (10 alike) : Product  RndMeth=Zero
  Product12 : Product  Inputs=3  RndMeth=Zero
  Product13 : Product  Inputs=3  RndMeth=Zero
  Sat(x) : Lookup_n-D  NumberOfTableDimensions=1  BreakpointsForDimension1=xVec  Table=SatX  InternalRulePriority=Speed  RndMeth=Simplest  InputSameDT=on
  Subtract1 : Sum  Inputs=++-
  Subtract11 : Sum  Inputs=+-
  Subtract12 : Sum  Inputs=+---
  Subtract13 : Sum  Inputs=+-+-
  Subtract14 : Sum
  Subtract15 : Sum  Inputs=--
  Subtract16 : Sum  Inputs=-+
  Subtract17 : Sum  Inputs=-+
  Subtract18 : Sum
  Subtract19 : Sum
  Subtract2 : Sum  Inputs=-+-
  Subtract3 : Sum  Inputs=+-
  Subtract4 : Sum  Inputs=-++
  Switch : Switch  Criteria=u2 > Threshold  Threshold=0.5
  fun : Fcn  Expr=u(1)/(u(2)+eps)
  fun1 : Fcn  Expr=u(1)/(u(2)+eps)
  gain3 : Gain  Gain=Kis
  gain4 : Gain  Gain=Xl
  gain5 : Gain  Gain=Xl
  psi_ag : Fcn  Expr=sqrt( (u(1)+Ra*u(3)+Xl*u(4))^2+(u(2)+Ra*u(4)-Xl*u(3))^2 )
  I : Outport  VectorParamsAs1DForOutWhenUnconnected=off
  Te : Outport  Port=2  VectorParamsAs1DForOutWhenUnconnected=off
  phimqd : Outport  Port=3  VectorParamsAs1DForOutWhenUnconnected=off
  Lmqd : Outport  Port=4  VectorParamsAs1DForOutWhenUnconnected=off
  wires:
  Switch/1 -> Bias2/1, Gain10/1
  Sat(x)/1 -> Switch/1
  Constant1/1 -> Switch/3
  Constant/1 -> Switch/2
  Product2/1 -> Gain4/1, Subtract2/1
  Gain8/1 -> Subtract3/2
  [Sat_d] -> Product2/1  "Sat_d"
  [wrpu] -> Product6/2  "1+w"
  Eqp/1 -> Product1/1  "Eqp"
  Gain2/1 -> Eqp/1
  Gain/1 -> Eqpp/1
  [Sat_d] -> Product1/2  "Sat_d"
  Gain1/1 -> Subtract2/3
  Eqpp/1 -> Product2/2, Product6/1, [Eqpp]  "Eqpp"
  Gain4/1 -> Subtract11/2, Subtract1/1
  [wrpu] -> Product7/2  "1+w"
  Efd/1 -> Subtract1/2  "Efd"
  [Sat_q] -> Product4/2  "Sat_q"
  Product5/1 -> Subtract4/1, Gain9/1
  Edpp/1 -> Product5/2, Product7/1, [Edpp]  "Edpp"
  Gain7/1 -> Edp/1
  Gain5/1 -> Edpp/1
  Gain6/1 -> Subtract4/3
  Subtract4/1 -> Gain5/1
  Subtract3/1 -> Gain7/1
  Subtract1/1 -> Gain2/1
  Product4/1 -> Gain8/1, Subtract4/2
  [id] -> Gain1/1  "id"
  Gain3/1 -> Subtract11/1, Subtract1/3
  Edp/1 -> Product4/1  "Edp"
  Product1/1 -> Subtract2/2, Gain3/1
  Gain9/1 -> Subtract3/1
  [iq] -> Gain6/1  "iq"
  [Sat_q] -> Product5/1  "Sat_q"
  Subtract2/1 -> Gain/1
  vqdTer/1 -> [vqdTer]
  wrpu/1 -> [wrpu]
  Subtract11/1 -> [ifd]
  Product6/1 -> [vq]  "vq"
  Product7/1 -> [vd]  "vd"
  [iq] -> Mux5/1
  [id] -> Mux5/2
  Mux5/1 -> I/1
  [Sat_q] -> Fcn3/1
  [Sat_d] -> Fcn2/1
  Fcn3/1 -> Mux6/1
  Fcn2/1 -> Mux6/2
  Mux6/1 -> Lmqd/1
  [ifd] -> Mux5/3
  Subtract17/1 -> Te/1
  Product3/1 -> Subtract17/1
  Product16/1 -> Subtract17/2
  [iq] -> Product16/1
  [id] -> Product3/1
  [Eqpp] -> Subtract16/2
  Product15/1 -> Subtract16/1
  [Edpp] -> Subtract15/2
  Product14/1 -> Subtract15/1
  Math Function1/1 -> gain3/1
  Bias2/1 -> [Sat_d]
  Bias3/1 -> [Sat_q]
  Gain10/1 -> Bias3/1
  Mux10/1 -> psi_ag/1
  psi_ag/1 -> Subtract14/1
  gain3/1 -> Subtract14/2
  Fcn5/1 -> [Xqsatpp]  "Xqsatpp"
  Fcn4/1 -> [Xdsatpp]  "Xdsatpp"
  [Sat_q] -> Fcn5/1  "Sat_q"
  [Sat_d] -> Fcn4/1  "Sat_d"
  Subtract14/1 -> Sat(x)/1
  [iq] -> Product14/1
  [Xqsatpp] -> Product14/2
  [id] -> Product15/1
  [Xdsatpp] -> Product15/2
  [id] -> Math Function1/2, Mux10/3
  [iq] -> Mux10/2, Math Function1/1
  [vqdTer] -> Demux4/1
  Subtract12/1 -> Gain17/1
  Iq/1 -> [iq], Gain15/1
  Demux4/1 -> [vqTer]
  Demux4/2 -> [vdTer]
  [vq] -> Subtract12/1
  [vqTer] -> Subtract12/2
  Gain15/1 -> Subtract12/4
  Subtract13/1 -> Gain18/1
  Id/1 -> Gain16/1, [id]
  [vd] -> Subtract13/1
  [vdTer] -> Subtract13/2
  Gain16/1 -> Subtract13/4
  [id] -> Product12/1
  [Xdsatpp] -> Product12/2
  Product12/1 -> Subtract12/3
  [iq] -> Product13/1
  [Xqsatpp] -> Product13/2
  Product13/1 -> Subtract13/3
  [wrpu] -> Product12/3
  [wrpu] -> Product13/3
  Mux8/1 -> fun/1
  Gain17/1 -> Mux8/1
  [Xqsatpp] -> Mux8/2
  fun/1 -> Iq/1
  Mux9/1 -> fun1/1
  Gain18/1 -> Mux9/1
  [Xdsatpp] -> Mux9/2
  fun1/1 -> Id/1
  [vqdTer] -> Mux10/1
  Subtract16/1 -> Subtract18/1, Product16/2
  Subtract15/1 -> Subtract19/1, Product3/2
  [iq] -> gain4/1
  gain4/1 -> Subtract19/2
  [id] -> gain5/1
  gain5/1 -> Subtract18/2
  Subtract19/1 -> Mux12/1
  Subtract18/1 -> Mux12/2
  Mux12/1 -> phimqd/1

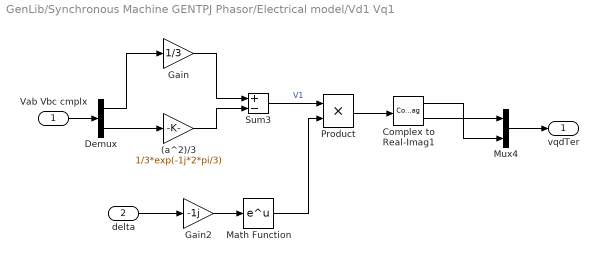
== system GenLib/Synchronous Machine GENTPJ Phasor/Electrical model/Vd1 Vq1 ==
  Vab Vbc cmplx : Inport
  delta : Inport  Port=2
  (a^2)/3 : Gain  Gain=1/3*exp(-1j*2*pi/3)  SaturateOnIntegerOverflow=on  OutDataTypeStr=Inherit: Same as input  ParamDataTypeStr=Inherit: Same as input
  Complex to Real-Imag1 : ComplexToRealImag
  Demux : Demux  Outputs=2
  Gain : Gain  Gain=1/3  SaturateOnIntegerOverflow=on  OutDataTypeStr=Inherit: Same as input  ParamDataTypeStr=Inherit: Same as input
  Gain2 : Gain  Gain=-1j  SaturateOnIntegerOverflow=on  OutDataTypeStr=Inherit: Same as input  ParamDataTypeStr=Inherit: Same as input
  Math Function : Math  SaturateOnIntegerOverflow=on
  Mux4 : Mux  Inputs=2
  Product : Product  SaturateOnIntegerOverflow=on  InputSameDT=on  OutDataTypeStr=Inherit: Same as first input
  Sum3 : Sum  Inputs=+-  SaturateOnIntegerOverflow=on  InputSameDT=on  OutDataTypeStr=Inherit: Same as first input
  vqdTer : Outport  VectorParamsAs1DForOutWhenUnconnected=off
  wires:
  delta/1 -> Gain2/1
  Demux/1 -> Gain/1
  Vab Vbc cmplx/1 -> Demux/1
  Gain/1 -> Sum3/1
  Sum3/1 -> Product/1  "V1"
  Complex to Real-Imag1/2 -> Mux4/1
  Complex to Real-Imag1/1 -> Mux4/2
  Demux/2 -> (a^2)/3/1
  (a^2)/3/1 -> Sum3/2
  Gain2/1 -> Math Function/1
  Product/1 -> Complex to Real-Imag1/1
  Math Function/1 -> Product/2
  Mux4/1 -> vqdTer/1

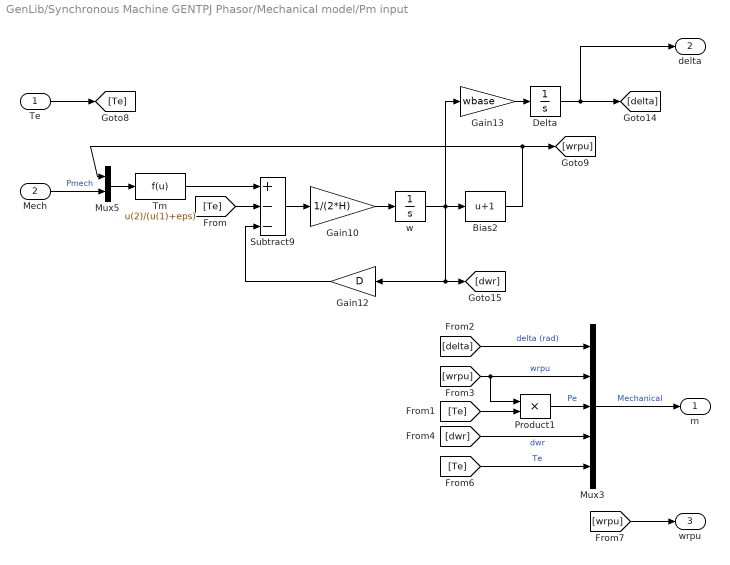
== system GenLib/Synchronous Machine GENTPJ Phasor/Mechanical model/Pm input ==
  Te : Inport
  Mech : Inport  Port=2
  Bias2 : Bias  Bias=1
  Delta : Integrator
  Gain10 : Gain  Gain=1/(2*H)
  Gain12 : Gain  Gain=D
  Gain13 : Gain  Gain=wbase
  Mux3 : Mux  Inputs=[1,1,1,1,1]
  Mux5 : Mux  Inputs=2
  Product1 : Product  SaturateOnIntegerOverflow=on  InputSameDT=on  OutDataTypeStr=Inherit: Same as first input
  Subtract9 : Sum  Inputs=+--
  Tm : Fcn  Expr=u(2)/(u(1)+eps)
  w : Integrator
  m : Outport  VectorParamsAs1DForOutWhenUnconnected=off
  delta : Outport  Port=2  VectorParamsAs1DForOutWhenUnconnected=off
  wrpu : Outport  Port=3  VectorParamsAs1DForOutWhenUnconnected=off
  wires:
  Mech/1 -> Mux5/2  "Pmech"
  Tm/1 -> Subtract9/1
  Delta/1 -> [delta], delta/1
  Bias2/1 -> Mux5/1, [wrpu]
  Gain13/1 -> Delta/1
  Mux5/1 -> Tm/1
  Gain12/1 -> Subtract9/3
  w/1 -> Bias2/1, Gain12/1, [dwr], Gain13/1
  Gain10/1 -> w/1
  Subtract9/1 -> Gain10/1
  Te/1 -> [Te]
  [Te] -> Subtract9/2
  [delta] -> Mux3/1  "delta (rad)"
  [wrpu] -> Mux3/2, Product1/1  "wrpu"
  [Te] -> Product1/2
  Product1/1 -> Mux3/3  "Pe"
  [dwr] -> Mux3/4  "dwr"
  [Te] -> Mux3/5  "Te"
  Mux3/1 -> m/1  "Mechanical"
  [wrpu] -> wrpu/1

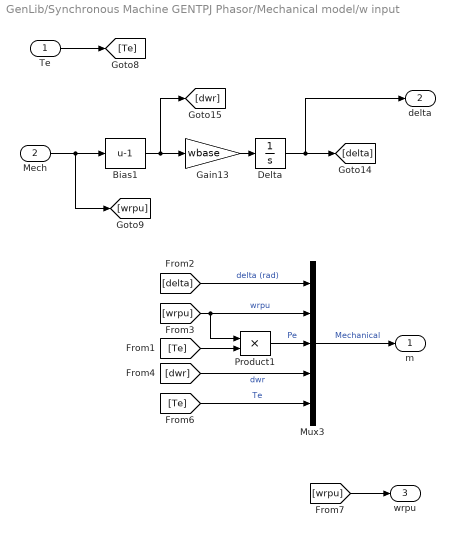
== system GenLib/Synchronous Machine GENTPJ Phasor/Mechanical model/w input ==
  Te : Inport
  Mech : Inport  Port=2
  Bias1 : Bias  Bias=-1
  Delta : Integrator
  Gain13 : Gain  Gain=wbase
  Mux3 : Mux  Inputs=[1,1,1,1,1]
  Product1 : Product  SaturateOnIntegerOverflow=on  InputSameDT=on  OutDataTypeStr=Inherit: Same as first input
  m : Outport  VectorParamsAs1DForOutWhenUnconnected=off
  delta : Outport  Port=2  VectorParamsAs1DForOutWhenUnconnected=off
  wrpu : Outport  Port=3  VectorParamsAs1DForOutWhenUnconnected=off
  wires:
  Bias1/1 -> Gain13/1, [dwr]
  Mech/1 -> [wrpu], Bias1/1
  Delta/1 -> [delta], delta/1
  Gain13/1 -> Delta/1
  Te/1 -> [Te]
  [delta] -> Mux3/1  "delta (rad)"
  [wrpu] -> Mux3/2, Product1/1  "wrpu"
  [Te] -> Product1/2
  Product1/1 -> Mux3/3  "Pe"
  [dwr] -> Mux3/4  "dwr"
  [Te] -> Mux3/5  "Te"
  Mux3/1 -> m/1  "Mechanical"
  [wrpu] -> wrpu/1

== system GenLib/Three-Phase Dynamic Load (custom)/Model/Break Alg. Loop I1 ==
  In : Inport
  Complex to Real-Imag : ComplexToRealImag
  Real-Imag to Complex : RealImagToComplex
  imag : Subsystem  mask(Transfer Function with Initial Outputs){N=[1], D=[5e-3  1], Y0=real(I1_init), U0=real(I1_init)}
      mask prompts: N "Numerator:"; D "Denominator:"; Y0 "Initial output:"; U0 "Initial input:"
      mask help: Vector expressions for numerator, and denominator. Coefficients are in descending powers of s.
      mask init:
      | [A,B,C,Dd]=tf2ss(N,D);if (isempty(Y0));[m,n]=size(A);X0=zeros(1,m); end; if (isempty(U0));[m,p]=size(B);U0=zeros(1,p);end;X0=getxo(A,B,C,Dd,U0,Y0,0);
      mask Help: Specify the initial output for the transfer function.  An optimization routine attempts to determine the appropriate initial states so that the specified initial output is achieved.  For more details, see the m-file getxo.m
      mask Display: dpoly(N,D,'s')
  real : Subsystem  mask(Transfer Function with Initial Outputs){N=[1], D=[5e-3  1], Y0=real(I1_init), U0=real(I1_init)}
      mask prompts: N "Numerator:"; D "Denominator:"; Y0 "Initial output:"; U0 "Initial input:"
      mask help: Vector expressions for numerator, and denominator. Coefficients are in descending powers of s.
      mask init:
      | [A,B,C,Dd]=tf2ss(N,D);if (isempty(Y0));[m,n]=size(A);X0=zeros(1,m); end; if (isempty(U0));[m,p]=size(B);U0=zeros(1,p);end;X0=getxo(A,B,C,Dd,U0,Y0,0);
      mask Help: Specify the initial output for the transfer function.  An optimization routine attempts to determine the appropriate initial states so that the specified initial output is achieved.  For more details, see the m-file getxo.m
      mask Display: dpoly(N,D,'s')
  Out : Outport  VectorParamsAs1DForOutWhenUnconnected=off
  wires:
  imag/1(Out1) -> Real-Imag to Complex/2
  Complex to Real-Imag/2 -> imag/1(In1)
  real/1(Out1) -> Real-Imag to Complex/1
  Complex to Real-Imag/1 -> real/1(In1)
  Real-Imag to Complex/1 -> Out/1
  In/1 -> Complex to Real-Imag/1

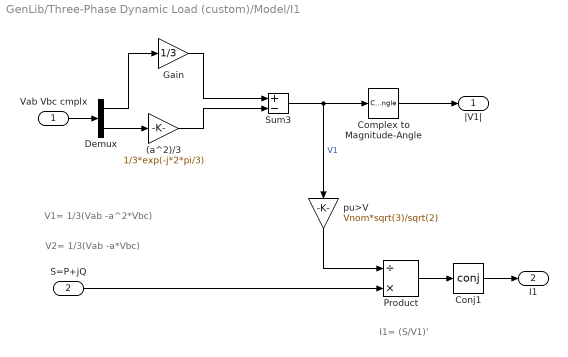
== system GenLib/Three-Phase Dynamic Load (custom)/Model/I1  ==
  note: V2= 1/3(Vab -a*Vbc)
  note: V1= 1/3(Vab -a^2*Vbc)
  note: I1= (S/V1)'
  Vab Vbc cmplx : Inport
  S=P+jQ : Inport  Port=2
  (a^2)/3 : Gain  Gain=1/3*exp(-j*2*pi/3)  SaturateOnIntegerOverflow=on  OutDataTypeStr=Inherit: Same as input  ParamDataTypeStr=Inherit: Same as input
  Complex to Magnitude-Angle : ComplexToMagnitudeAngle  Output=Magnitude
  Conj1 : Math  Operator=conj  SaturateOnIntegerOverflow=on
  Demux : Demux  Outputs=2
  Gain : Gain  Gain=1/3  SaturateOnIntegerOverflow=on  OutDataTypeStr=Inherit: Same as input  ParamDataTypeStr=Inherit: Same as input
  Product : Product  Inputs=/*  SaturateOnIntegerOverflow=on  InputSameDT=on  OutDataTypeStr=Inherit: Same as first input
  Sum3 : Sum  Inputs=+-  SaturateOnIntegerOverflow=on  InputSameDT=on  OutDataTypeStr=Inherit: Same as first input
  pu>V : Gain  Gain=Vnom*sqrt(3)/sqrt(2)  SaturateOnIntegerOverflow=on  OutDataTypeStr=Inherit: Same as input  ParamDataTypeStr=Inherit: Same as input
  |V1| : Outport  VectorParamsAs1DForOutWhenUnconnected=off
  I1 : Outport  Port=2  VectorParamsAs1DForOutWhenUnconnected=off
  wires:
  (a^2)/3/1 -> Sum3/2
  Demux/2 -> (a^2)/3/1
  Gain/1 -> Sum3/1
  Vab Vbc cmplx/1 -> Demux/1
  Demux/1 -> Gain/1
  Sum3/1 -> Complex to Magnitude-Angle/1, pu>V/1  "V1"
  Complex to Magnitude-Angle/1 -> |V1|/1
  S=P+jQ/1 -> Product/2
  Product/1 -> Conj1/1
  Conj1/1 -> I1/1
  pu>V/1 -> Product/1

== system GenLib/Three-Phase Dynamic Load (custom)/Model/Phase currents ==
  note: Ib= a^2*I1
  note: Ia= I1
  I1 : Inport
  Mux1 : Mux  Inputs=2
  a^2 : Gain  Gain=exp(-j*2*pi/3)  SaturateOnIntegerOverflow=on  OutDataTypeStr=Inherit: Same as input  ParamDataTypeStr=Inherit: Same as input
  Ia Ib cmplx : Outport  VectorParamsAs1DForOutWhenUnconnected=off
  wires:
  Mux1/1 -> Ia Ib cmplx/1  "ia ib"
  I1/1 -> a^2/1, Mux1/1
  a^2/1 -> Mux1/2

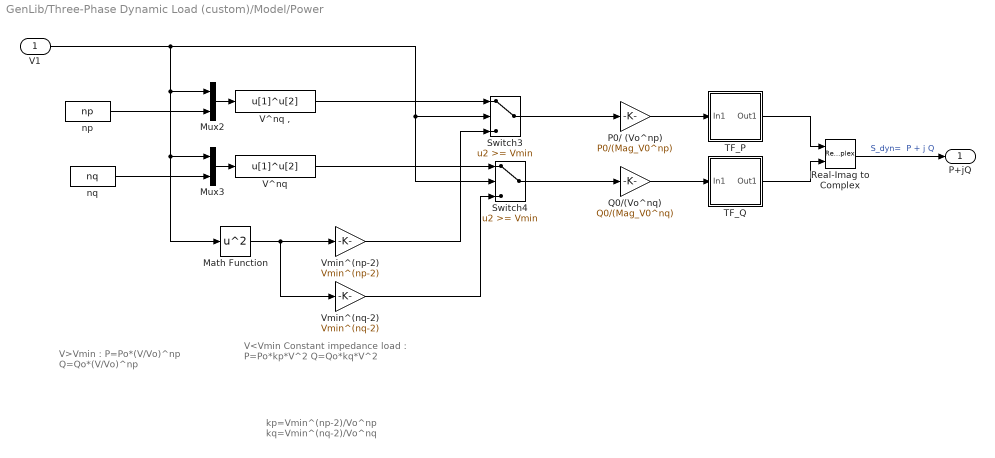
== system GenLib/Three-Phase Dynamic Load (custom)/Model/Power ==
  note: V>Vmin :
      |
      |    P=Po*(V/Vo)^np
      |    Q=Qo*(V/Vo)^np
  note: V<Vmin
      | Constant impedance load :
      |
      |  P=Po*kp*V^2
      | Q=Qo*kq*V^2
  note: kp=Vmin^(np-2)/Vo^np
      | kq=Vmin^(nq-2)/Vo^nq
  V1 : Inport
  Math Function : Math  Operator=square  SaturateOnIntegerOverflow=on
  Mux2 : Mux  Inputs=2
  Mux3 : Mux  Inputs=2
  P0/ (Vo^np) : Gain  Gain=P0/(Mag_V0^np)  SaturateOnIntegerOverflow=on  OutDataTypeStr=Inherit: Same as input  ParamDataTypeStr=Inherit: Same as input
  Q0/(Vo^nq) : Gain  Gain=Q0/(Mag_V0^nq)  SaturateOnIntegerOverflow=on  OutDataTypeStr=Inherit: Same as input  ParamDataTypeStr=Inherit: Same as input
  Real-Imag to Complex : RealImagToComplex
  Switch3 : Switch  Threshold=Vmin  InputSameDT=on
  Switch4 : Switch  Threshold=Vmin  InputSameDT=on
  TF_P : Subsystem  mask(Transfer function){T1=Tp1, T2=Tp2, V_Init=P0}
      mask prompts: T1 "Time constant T1 (s):"; T2 "Time constant T2 (s):"; V_Init "Initial input and output :"
      mask help:
      | This block implements a continuous transfer function:
      |
      |          1+T1s
      | H(s)= ------
      |          1+T2s
      |
      | States are initialized according to  initial input and output value so that simulation starts in steady state.
      mask init:
      | numc=[T1 1];
      | denc=[T2 1];
      | [Ac,Bc,Cc,Dc]=tf2ss(numc,denc);
      | 
      | % Compute Initial states
      | I=eye(size(Ac));
      | x0c=inv(-Ac)*Bc*V_Init;
      mask Display: disp('1+T1s\n---\n1+T2s')
  TF_Q : Subsystem  mask(Transfer function){T1=Tq1, T2=Tq2, V_Init=Q0}
      mask prompts: T1 "Time constant T1 (s):"; T2 "Time constant T2 (s):"; V_Init "Initial input and output :"
      mask help:
      | This block implements a continuous transfer function:
      |
      |          1+T1s
      | H(s)= ------
      |          1+T2s
      |
      | States are initialized according to  initial input and output value so that simulation starts in steady state.
      mask init:
      | numc=[T1 1];
      | denc=[T2 1];
      | [Ac,Bc,Cc,Dc]=tf2ss(numc,denc);
      | 
      | % Compute Initial states
      | I=eye(size(Ac));
      | x0c=inv(-Ac)*Bc*V_Init;
      mask Display: disp('1+T1s\n---\n1+T2s')
  V^nq : Fcn  Expr=u[1]^u[2]
  V^nq , : Fcn  Expr=u[1]^u[2]
  Vmin^(np-2) : Gain  Gain=Vmin^(np-2)  SaturateOnIntegerOverflow=on  OutDataTypeStr=Inherit: Same as input  ParamDataTypeStr=Inherit: Same as input
  Vmin^(nq-2) : Gain  Gain=Vmin^(nq-2)  SaturateOnIntegerOverflow=on  OutDataTypeStr=Inherit: Same as input  ParamDataTypeStr=Inherit: Same as input
  np : Constant  Value=np
  nq : Constant  Value=nq
  P+jQ : Outport  VectorParamsAs1DForOutWhenUnconnected=off
  wires:
  Switch4/1 -> Q0/(Vo^nq)/1
  Real-Imag to Complex/1 -> P+jQ/1  "S_dyn=  P + j Q"
  P0/ (Vo^np)/1 -> TF_P/1(In1)
  Q0/(Vo^nq)/1 -> TF_Q/1(In1)
  Switch3/1 -> P0/ (Vo^np)/1
  np/1 -> Mux2/2
  Mux2/1 -> V^nq ,/1
  nq/1 -> Mux3/2
  Mux3/1 -> V^nq/1
  V1/1 -> Mux2/1, Mux3/1, Math Function/1, Switch3/2, Switch4/2
  V^nq/1 -> Switch4/1
  Math Function/1 -> Vmin^(np-2)/1, Vmin^(nq-2)/1
  Vmin^(np-2)/1 -> Switch3/3
  V^nq ,/1 -> Switch3/1
  Vmin^(nq-2)/1 -> Switch4/3
  TF_P/1(Out1) -> Real-Imag to Complex/1
  TF_Q/1(Out1) -> Real-Imag to Complex/2

== system GenLib/Synchronous Machine GENTPJ Phasor/Electrical model/Machine measurements/Delta angle ==
  Vqd : Inport
  Complex to Magnitude-Angle : ComplexToMagnitudeAngle  Output=Angle
  Demux1 : Demux  Outputs=2
  Real-Imag to Complex : RealImagToComplex
  rad2deg : Gain  Gain=180/pi
  delta : Outport  VectorParamsAs1DForOutWhenUnconnected=off
  wires:
  Vqd/1 -> Demux1/1
  rad2deg/1 -> delta/1
  Demux1/2 -> Real-Imag to Complex/2
  Demux1/1 -> Real-Imag to Complex/1
  Real-Imag to Complex/1 -> Complex to Magnitude-Angle/1
  Complex to Magnitude-Angle/1 -> rad2deg/1

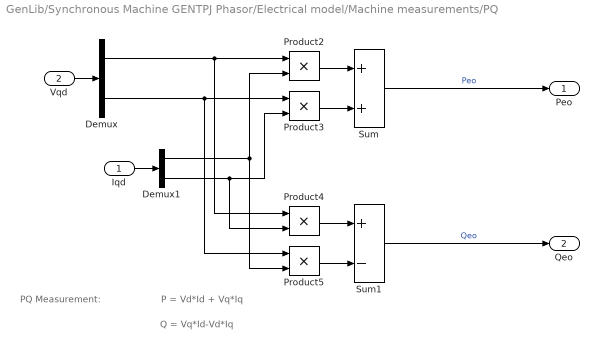
== system GenLib/Synchronous Machine GENTPJ Phasor/Electrical model/Machine measurements/PQ ==
  note: PQ Measurement:
  note: Q = Vq*Id-Vd*Iq
  note: P = Vd*Id + Vq*Iq
  Iqd : Inport
  Vqd : Inport  Port=2
  Demux : Demux  Outputs=2
  Demux1 : Demux  Outputs=[1,1]
  Product{2..5} (4 alike) : Product  SaturateOnIntegerOverflow=on  InputSameDT=on  OutDataTypeStr=Inherit: Same as first input
  Sum : Sum  SaturateOnIntegerOverflow=on  InputSameDT=on  OutDataTypeStr=Inherit: Same as first input
  Sum1 : Sum  Inputs=+-  SaturateOnIntegerOverflow=on  InputSameDT=on  OutDataTypeStr=Inherit: Same as first input
  Peo : Outport  VectorParamsAs1DForOutWhenUnconnected=off
  Qeo : Outport  Port=2  VectorParamsAs1DForOutWhenUnconnected=off
  wires:
  Demux1/2 -> Product4/2, Product3/2
  Demux/1 -> Product4/1, Product2/1
  Demux/2 -> Product5/1, Product3/1
  Sum1/1 -> Qeo/1  "Qeo"
  Sum/1 -> Peo/1  "Peo"
  Product5/1 -> Sum1/2
  Product4/1 -> Sum1/1
  Product3/1 -> Sum/2
  Product2/1 -> Sum/1
  Iqd/1 -> Demux1/1
  Demux1/1 -> Product2/2, Product5/2
  Vqd/1 -> Demux/1

== system GenLib/Three-Phase Dynamic Load (custom)/Model/Break Alg. Loop I1/imag ==
  In1 : Inport
  State Space : StateSpace  A=A  B=B  C=C  D=Dd  InitialCondition=X0
  Out1 : Outport  InitialOutput=0  VectorParamsAs1DForOutWhenUnconnected=off
  wires:
  State Space/1 -> Out1/1
  In1/1 -> State Space/1

== system GenLib/Three-Phase Dynamic Load (custom)/Model/Break Alg. Loop I1/real ==
  In1 : Inport
  State Space : StateSpace  A=A  B=B  C=C  D=Dd  InitialCondition=X0
  Out1 : Outport  InitialOutput=0  VectorParamsAs1DForOutWhenUnconnected=off
  wires:
  In1/1 -> State Space/1
  State Space/1 -> Out1/1

== system GenLib/Three-Phase Dynamic Load (custom)/Model/Power/TF_P ==
  In1 : Inport
  State-Space : StateSpace  A=Ac  B=Bc  C=Cc  D=Dc  InitialCondition=x0c
  Out1 : Outport  VectorParamsAs1DForOutWhenUnconnected=off
  wires:
  State-Space/1 -> Out1/1
  In1/1 -> State-Space/1

== system GenLib/Three-Phase Dynamic Load (custom)/Model/Power/TF_Q ==
  In1 : Inport
  State-Space : StateSpace  A=Ac  B=Bc  C=Cc  D=Dc  InitialCondition=x0c
  Out1 : Outport  VectorParamsAs1DForOutWhenUnconnected=off
  wires:
  In1/1 -> State-Space/1
  State-Space/1 -> Out1/1
